simulink model "BandPassFilterModel1"  (R2021a)
settings: Solver=VariableStepAuto  StartTime=0.0  StopTime=10.0  RelTol=1e-3
settings Model: Creator=asus  LastModifiedBy=asus

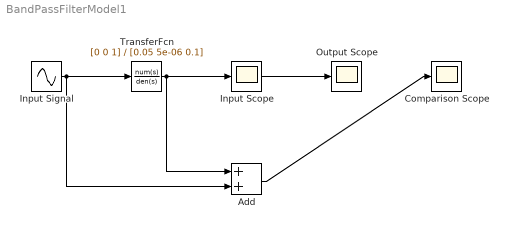
== system BandPassFilterModel1 ==
  Add : Sum
  Comparison Scope : Scope
  Input Scope : Scope
  Input Signal : Sin  SampleTime=0
  Output Scope : Scope
  TransferFcn : TransferFcn  Numerator=[0 0 1]  Denominator=[0.05 5e-06 0.1]
  wires:
  Input Signal/1 -> TransferFcn/1, Input Scope/1, Add/2
  TransferFcn/1 -> Output Scope/1, Add/1
  Add/1 -> Comparison Scope/1
